simulink model "c2_3zhuangtaifankui"  (R2019b)
settings: Solver=VariableStepAuto  StartTime=0.0  StopTime=40  RelTol=1e-3
settings Model: Creator=MAY  LastModifiedBy=wy151
settings DataIOCC: ReturnWorkspaceOutputs=off
settings OptimizationCC: LifeSpan=inf
settings DebuggingCC: SFExecutionAtInitializationDiag=none  ArithmeticOperatorsInVariantConditions=warning
settings SFSimCC: SimUseLocalCustomCode=off  CustomCodeUndefinedFunction=UseInterfaceOnly
settings RTWCC: RTWUseLocalCustomCode=off
settings CodeAppCC: StateflowObjectComments=on
settings SimscapeCC: SimscapeNormalizeSystem=off

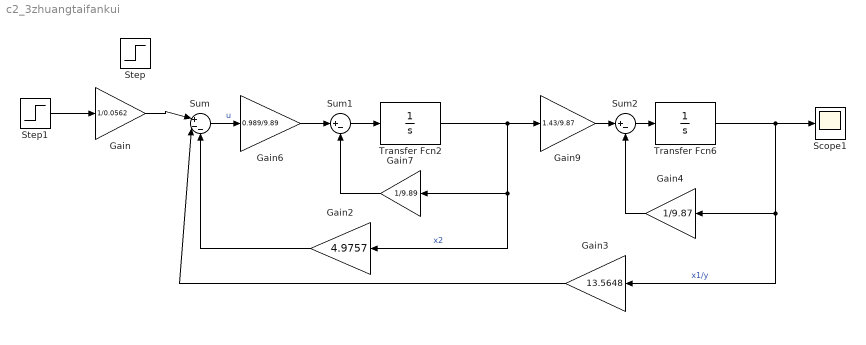
== system c2_3zhuangtaifankui ==
  Gain : Gain  Gain=1/0.0562
  Gain2 : Gain  Gain=4.9757
  Gain3 : Gain  Gain=13.5648
  Gain4 : Gain  Gain=1/9.87
  Gain6 : Gain  Gain=0.989/9.89
  Gain7 : Gain  Gain=1/9.89
  Gain9 : Gain  Gain=1.43/9.87
  Scope1 : Scope
  Step : Step  SampleTime=0
  Step1 : Step  SampleTime=0
  Sum : Sum  Inputs=|+--
  Sum1 : Sum  Inputs=|+-
  Sum2 : Sum  Inputs=|+-
  Transfer Fcn2 : TransferFcn  Denominator=[1 0]
  Transfer Fcn6 : TransferFcn  Denominator=[1 0]
  wires:
  Sum/1 -> Gain6/1  "u"
  Step1/1 -> Gain/1
  Gain7/1 -> Sum1/2
  Sum1/1 -> Transfer Fcn2/1
  Gain6/1 -> Sum1/1
  Transfer Fcn2/1 -> Gain9/1, Gain2/1, Gain7/1  "x2"
  Transfer Fcn6/1 -> Scope1/1, Gain3/1, Gain4/1  "x1/y"
  Gain9/1 -> Sum2/1
  Sum2/1 -> Transfer Fcn6/1
  Gain4/1 -> Sum2/2
  Gain2/1 -> Sum/3
  Gain3/1 -> Sum/2
  Gain/1 -> Sum/1
